simulink model "lookup_nD_TestGen22"  (R2017b)
settings: Solver=FixedStepDiscrete  StartTime=0.0  StopTime=10.0  RelTol=1e-3
settings Model: Creator=ktrinh  LastModifiedBy=ktrinh
settings DebuggingCC: ParameterOverflowMsg=none

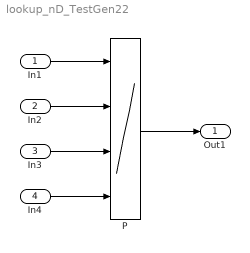
== system lookup_nD_TestGen22 ==
  In1 : Inport  OutMin=0  OutMax=127  PortDimensions=1
  In2 : Inport  Port=2  OutMin=0  OutMax=127
  In3 : Inport  Port=3  OutMin=0  OutMax=127
  In4 : Inport  Port=4  OutMin=0  OutMax=127
  P : Lookup_n-D  NumberOfTableDimensions=4  BreakpointsSpecification=Even spacing  BreakpointsForDimension3=[5, 7]  BreakpointsForDimension1FirstPoint=50.8813  BreakpointsForDimension2FirstPoint=47.8707  BreakpointsForDimension3FirstPoint=42.1635  BreakpointsForDimension4FirstPoint=93.1291  BreakpointsForDimension1Spacing=1.5  BreakpointsForDimension2Spacing=1.5  BreakpointsForDimension3Spacing=1.5  BreakpointsForDimension4Spacing=1.5  Table=reshape(repmat([4 5 6 7 8;16 19 20 21 22;10 18 23 24 25],2,2),[2,5,3,2])  InterpMethod=Nearest  InternalRulePriority=Speed  RndMeth=Simplest  InputSameDT=on
  Out1 : Outport
  wires:
  In1/1 -> P/1
  In2/1 -> P/2
  In3/1 -> P/3
  In4/1 -> P/4
  P/1 -> Out1/1
